simulink model "Question2"  (R2018a)
settings: Solver=VariableStepDiscrete  StartTime=0.0  StopTime=0.5  RelTol=1e-3
libraries: powerlib x10, powerlib_meascontrol x1, dspstat3 x1
settings Model: Creator=enes_  LastModifiedBy=enes_

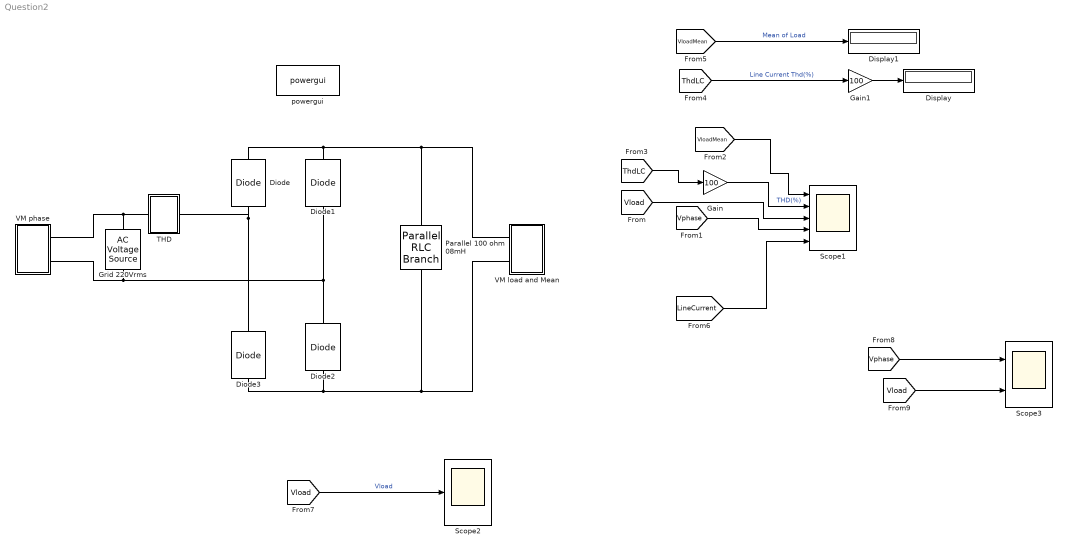
== system Question2 ==
  Diode{,1..3} (4 alike) : powerlib/Power Electronics/Diode  Ron=0.001  Lon=0  Vf=0.8  IC=0  UseSnubber=0  Rs=500  Cs=250e-9  Measurements=off
  Display : Display
  Display1 : Display
  Gain : Gain  Gain=100
  Gain1 : Gain  Gain=100
  Grid 220Vrms : powerlib/Electrical Sources/AC Voltage Source  Amplitude=326.6  Phase=0  Frequency=50  SampleTime=0  Measurements=None  BusType=swing  Pref=10e3  Qref=0  Qmin=-inf  Qmax=+inf
  Parallel 100 ohm 08mH : powerlib/Elements/Parallel RLC Branch  LConnTagsString=a  RConnTagsString=__new0  BranchType=RC  Resistance=100  Inductance=1e-3  SetiL0=off  InitialCurrent=0  Capacitance=0.8e-3  Setx0=off  InitialVoltage=0  Measurements=None
  Scope1 : Scope  NumInputPorts=5
  Scope2 : Scope
  Scope3 : Scope  NumInputPorts=2
  THD : Subsystem
  VM load and Mean : Subsystem
  VM phase : Subsystem
  powergui : powerlib/powergui  Priority=1  SimulationMode=Discrete  SampleTime=1e-6  frequency=60  Iterations=50  frequencyindice=50  Pbase=100e6  ErrMax=1e-4  UnitsV=kV  UnitsW=MW  buscounter=0  FunctionMessages=off  echomessages=off  EnableUseOfTLC=off  CurrentSourceSwitches=off  DisableSnubberDevices=off  DisableRonSwitches=off  DisableVfSwitches=off  DisplayEquations=off  SolverType=Tustin/Backward Euler (TBE)  Interpol=off  ExternalGateDelay=off  methode=off  Ts=100  x0status=blocks  SPID=on  SwTol=0  HookPort=off  RestoreLinks=warning  ResistiveCurrentMeasurement=off  Frange=[0:2:500]  Ylog=off  Xlog=on  ShowGrid=off  save=off  variable=ZData  structure=0  ZoomFFT=on  StartTime=0.0  cycles=1  DisplayStyle=1  fundamental=60  FreqAxis=off  MaxFrequency=1000  frequencyindicesteady=1  RmsSteady=1  display=off
  wires:
  [Vphase] -> Scope1/4
  [Vload] -> Scope1/3
  [VloadMean] -> Scope1/1
  [ThdLC] -> Gain1/1  "Line Current Thd(%)"
  [ThdLC] -> Gain/1
  Gain/1 -> Scope1/2  "THD(%)"
  [VloadMean] -> Display1/1  "Mean of Load"
  [LineCurrent] -> Scope1/5
  [Vload] -> Scope2/1  "Vload"
  Gain1/1 -> Display/1
  [Vload] -> Scope3/2
  [Vphase] -> Scope3/1
  connections:
  Diode1/RConn1 -- Parallel 100 ohm 08mH/LConn1 -- VM load and Mean/LConn1 -- Diode/RConn1
  VM load and Mean/LConn2 -- Diode2/LConn1 -- Diode3/LConn1 -- Parallel 100 ohm 08mH/RConn1
  Diode/LConn1 -- THD/RConn1 -- Diode3/RConn1
  Diode1/LConn1 -- Grid 220Vrms/LConn1 -- VM phase/LConn2 -- Diode2/RConn1
  Grid 220Vrms/RConn1 -- THD/LConn1 -- VM phase/LConn1

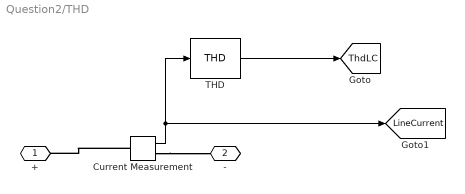
== system Question2/THD ==
  Current Measurement : powerlib/Measurements/Current Measurement  PhasorSimulation=off  OutputType=Complex  PSBequivalent=0
  THD : powerlib_meascontrol/Measurements/THD  Freq=50  Ts=1e-6
  + : PMIOPort  Side=Left
  - : PMIOPort  Port=2  Side=Right
  tag scope: LineCurrent=global, ThdLC=global
  wires:
  THD/1 -> [ThdLC]
  Current Measurement/1 -> [LineCurrent], THD/1
  connections:
  Current Measurement/RConn1 -- -/RConn1
  Current Measurement/LConn1 -- +/RConn1

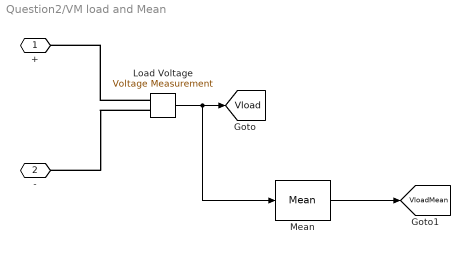
== system Question2/VM load and Mean ==
  Load Voltage : powerlib/Measurements/Voltage Measurement  PhasorSimulation=off  OutputType=Complex  PSBequivalent=0
  Mean : dspstat3/Mean  run=on  InputProcessing=Columns as channels (frame based)  reset_popup=None  directionMode=Each column  dimension=1  roiEnable=off  roiType=Rectangles  roiPortion=Entire ROI  roiOutput=Individual statistics for each ROI  roiFlag=off  roundingMode=Floor  overflowMode=off  outputDataTypeStr=Inherit: Same as accumulator  outputMin=[]  outputMax=[]  outputLastDataTypeStr=Inherit: Same as accumulator
  + : PMIOPort  Side=Left
  - : PMIOPort  Port=2  Side=Left
  tag scope: Vload=global, VloadMean=global
  wires:
  Load Voltage/1 -> Mean/1, [Vload]
  Mean/1 -> [VloadMean]
  connections:
  Load Voltage/LConn1 -- +/RConn1
  Load Voltage/LConn2 -- -/RConn1

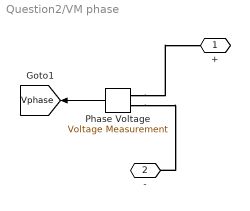
== system Question2/VM phase ==
  Phase Voltage : powerlib/Measurements/Voltage Measurement  PhasorSimulation=off  OutputType=Complex  PSBequivalent=0
  + : PMIOPort  Side=Left
  - : PMIOPort  Port=2  Side=Left
  tag scope: Vphase=global
  wires:
  Phase Voltage/1 -> [Vphase]
  connections:
  Phase Voltage/LConn1 -- +/RConn1
  Phase Voltage/LConn2 -- -/RConn1
